simulink model "PID_controller_long"  (R2019a)
settings: Solver=VariableStepAuto  StartTime=0.0  StopTime=100  FixedStep=1e-3  RelTol=1e-5
values from neighbouring files (symbols this model uses):
  sys = ss(A,B,C,D,'StateName', {'u'; 'w'; 'q'; 'theta'; 'h'}, 'InputName', {'eta';'epsilon'})    [control_system_v01.m]    (also in control_system_v02.m = ss(A,B,C,D,'StateName', {'u'; 'w'; 'q'; 'theta'},          ')
undefined symbols (not defined in the file or in its folder): a, actuators, b, c, env, F, geometry, Light, MIL
libraries: simulink x2, hdlsllib x1, aerolibactuator x1, aerolibwind2 x1, dspmtrx3 x1
settings Model: Creator=tyson  LastModifiedBy=tyson
settings DebuggingCC: InheritedTsInSrcMsg=none

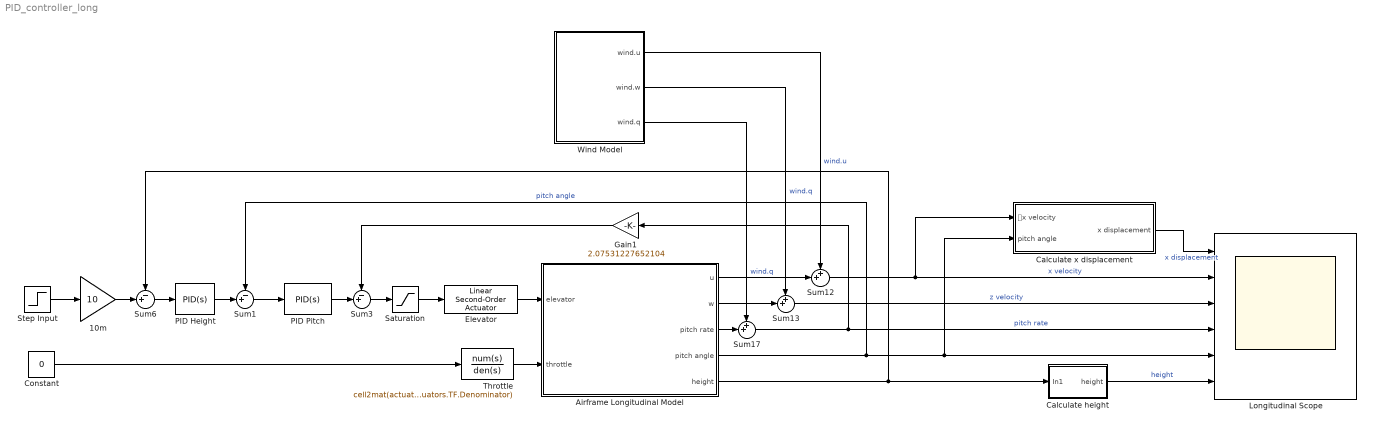
== system PID_controller_long ==
  10m : Gain  Gain=10
  Airframe Longitudinal Model : Subsystem
      mask Display: image('/home/tyson/Dropbox/Academic/4th Year/ELEN4011/matlab/icons/airframe_long.png');
  Calculate height : Subsystem
  Calculate x displacement : Subsystem
  Constant : Constant  Value=0
  Elevator : aerolibactuator/Linear Second-Order Actuator  wn_fin=actuators.naturalFreq  z_fin=actuators.dampingRatio  fin_act_0=0  fin_act_vel=0
      settings: SourceProductName=Aerospace Blockset  SourceProductBaseCode=AE
  Gain1 : Gain  Gain=2.07531227652104
  Longitudinal Scope : Scope  NumInputPorts=6
  PID Height : simulink/Continuous/PID Controller  Controller=PID  Form=Parallel  TimeDomain=Continuous-time  SampleTime=-1  IntegratorMethod=Forward Euler  FilterMethod=Forward Euler  ControllerParametersSource=internal  P=0.0203746551941326  I=3.98785899354423e-05  D=-0.014097541537027  UseFilter=on  N=1.21830283710381  TunerSelectOption=Transfer Function Based (PID Tuner App)  InitialConditionSource=internal  InitialConditionForIntegrator=0  InitialConditionForFilter=0  DifferentiatorICPrevScaledInput=0  ExternalReset=none  TrackingMode=off  Kt=1  LimitOutput=off  UpperSaturationLimit=deg2rad(12.5)  LowerSaturationLimit=-deg2rad(12.5)  LinearizeAsGain=on  AntiWindupMode=clamping  Kb=1  POutMin=[]  POutMax=[]  IOutMin=[]  IOutMax=[]  DOutMin=[]  DOutMax=[]  NOutMin=[]  NOutMax=[]  SumOutMin=[]  SumOutMax=[]  SaturationOutMin=[]  SaturationOutMax=[]  PParamMin=[]  PParamMax=[]  IParamMin=[]  IParamMax=[]  DParamMin=[]  DParamMax=[]  NParamMin=[]  NParamMax=[]  KbParamMin=[]  KbParamMax=[]  KtParamMin=[]  KtParamMax=[]  KbOutMin=[]  KbOutMax=[]  KtOutMin=[]  KtOutMax=[]  IntegratorOutMin=[]  IntegratorOutMax=[]  FilterOutMin=[]  FilterOutMax=[]  SumI1OutMin=[]  SumI1OutMax=[]  SumI2OutMin=[]  SumI2OutMax=[]  SumI3OutMin=[]  SumI3OutMax=[]  SumI4OutMin=[]  SumI4OutMax=[]  SumDOutMin=[]  SumDOutMax=[]  DifferentiatorOutMin=[]  DifferentiatorOutMax=[]  FilterDiffOutCoefMin=[]  FilterDiffOutCoefMax=[]  ReciprocalOutMin=[]  ReciprocalOutMax=[]  SumDenOutMin=[]  SumDenOutMax=[]  SumNumOutMin=[]  SumNumOutMax=[]  DivideOutMin=[]  DivideOutMax=[]  IntegratorContinuousStateAttributes=''  IntegratorStateMustResolveToSignalObject=off  IntegratorRTWStateStorageClass=Auto  FilterContinuousStateAttributes=''  FilterStateMustResolveToSignalObject=off  FilterRTWStateStorageClass=Auto  ParallelPVariant=InternalParameters  IdealPVariant=Disabled  IVariant=InternalParameters  DVariant=InternalParameters  IntegratorVariant=Continuous  SatVariant=Disabled  AWVariant=Passthrough  PCopyVariant=Disabled  TRVariant=Disabled  FdbkBlocksVariant=Forward  IdealPFdbkVariant=Disabled  SatFdbkVariant=Disabled  DerivativeFilterVariant=ContFilter  NVariant=InternalParameters  NCopyVariant=Disabled  FilterICVariant=InternalICsFilter  IntegratorICVariant=InternalICs  ExternalResetVariant=Disabled  TRSumVariant=Passthrough  SumFdbkVariant=Disabled  SumVariant=Sum_PID
  PID Pitch : simulink/Continuous/PID Controller  Controller=PID  Form=Parallel  TimeDomain=Continuous-time  SampleTime=-1  IntegratorMethod=Forward Euler  FilterMethod=Forward Euler  ControllerParametersSource=internal  P=11.4841294962751  I=3.73443810245113  D=6.13074519741651  UseFilter=on  N=502.258070962348  TunerSelectOption=Transfer Function Based (PID Tuner App)  InitialConditionSource=internal  InitialConditionForIntegrator=0  InitialConditionForFilter=0  DifferentiatorICPrevScaledInput=0  ExternalReset=none  TrackingMode=off  Kt=1  LimitOutput=on  UpperSaturationLimit=geometry.elevator.limits(1)  LowerSaturationLimit=geometry.elevator.limits(2)  LinearizeAsGain=on  AntiWindupMode=clamping  Kb=1  POutMin=[]  POutMax=[]  IOutMin=[]  IOutMax=[]  DOutMin=[]  DOutMax=[]  NOutMin=[]  NOutMax=[]  SumOutMin=[]  SumOutMax=[]  SaturationOutMin=[]  SaturationOutMax=[]  PParamMin=[]  PParamMax=[]  IParamMin=[]  IParamMax=[]  DParamMin=[]  DParamMax=[]  NParamMin=[]  NParamMax=[]  KbParamMin=[]  KbParamMax=[]  KtParamMin=[]  KtParamMax=[]  KbOutMin=[]  KbOutMax=[]  KtOutMin=[]  KtOutMax=[]  IntegratorOutMin=[]  IntegratorOutMax=[]  FilterOutMin=[]  FilterOutMax=[]  SumI1OutMin=[]  SumI1OutMax=[]  SumI2OutMin=[]  SumI2OutMax=[]  SumI3OutMin=[]  SumI3OutMax=[]  SumI4OutMin=[]  SumI4OutMax=[]  SumDOutMin=[]  SumDOutMax=[]  DifferentiatorOutMin=[]  DifferentiatorOutMax=[]  FilterDiffOutCoefMin=[]  FilterDiffOutCoefMax=[]  ReciprocalOutMin=[]  ReciprocalOutMax=[]  SumDenOutMin=[]  SumDenOutMax=[]  SumNumOutMin=[]  SumNumOutMax=[]  DivideOutMin=[]  DivideOutMax=[]  IntegratorContinuousStateAttributes=''  IntegratorStateMustResolveToSignalObject=off  IntegratorRTWStateStorageClass=Auto  FilterContinuousStateAttributes=''  FilterStateMustResolveToSignalObject=off  FilterRTWStateStorageClass=Auto  ParallelPVariant=InternalParameters  IdealPVariant=Disabled  IVariant=InternalParameters  DVariant=InternalParameters  IntegratorVariant=Continuous  SatVariant=Enabled  AWVariant=ContClampingParallel  PCopyVariant=Disabled  TRVariant=Disabled  FdbkBlocksVariant=Forward  IdealPFdbkVariant=Disabled  SatFdbkVariant=Disabled  DerivativeFilterVariant=ContFilter  NVariant=InternalParameters  NCopyVariant=Disabled  FilterICVariant=InternalICsFilter  IntegratorICVariant=InternalICs  ExternalResetVariant=Disabled  TRSumVariant=Passthrough  SumFdbkVariant=Disabled  SumVariant=Sum_PID
  Saturation : Saturate  UpperLimit=geometry.elevator.limits(1)  LowerLimit=geometry.elevator.limits(2)  LinearizeAsGain=off
  Step Input : Step  Time=0
  Sum1 : Sum  Inputs=-+|
  Sum12 : Sum  Inputs=++|
  Sum13 : Sum  Inputs=++|
  Sum17 : Sum  Inputs=++|
  Sum3 : Sum  Inputs=-+|
  Sum6 : Sum  Inputs=-+|
  Throttle : TransferFcn  Numerator=cell2mat(actuators.TF.Numerator)  Denominator=cell2mat(actuators.TF.Denominator)
  Wind Model : Subsystem
      mask Display: image('/home/tyson/Dropbox/Academic/4th Year/ELEN4011/matlab/icons/wind.png');
  wires:
  Airframe Longitudinal Model/4(pitch angle) -> Longitudinal Scope/5, Calculate x displacement/2(pitch angle), Sum1/1  "pitch angle"
  Sum13/1 -> Longitudinal Scope/3  "z velocity"
  Elevator/1 -> Airframe Longitudinal Model/1(elevator)
  Sum17/1 -> Longitudinal Scope/4, Gain1/1  "pitch rate"
  Sum1/1 -> PID Pitch/1
  PID Pitch/1 -> Sum3/2
  PID Height/1 -> Sum1/2
  Sum6/1 -> PID Height/1
  Sum3/1 -> Saturation/1
  Airframe Longitudinal Model/5(height) -> Calculate height/1(In1), Sum6/1
  Sum12/1 -> Calculate x displacement/1(𝚫x velocity), Longitudinal Scope/2  "x velocity"
  Calculate x displacement/1(x displacement) -> Longitudinal Scope/1  "x displacement"
  Airframe Longitudinal Model/1(u) -> Sum12/2
  Airframe Longitudinal Model/2(w) -> Sum13/2
  Airframe Longitudinal Model/3(pitch rate) -> Sum17/2
  Step Input/1 -> 10m/1
  10m/1 -> Sum6/2
  Wind Model/1(wind.u) -> Sum12/1  "wind.u"
  Wind Model/2(wind.w) -> Sum13/1  "wind.q"
  Wind Model/3(wind.q) -> Sum17/1  "wind.q"
  Throttle/1 -> Airframe Longitudinal Model/2(throttle)
  Gain1/1 -> Sum3/1
  Saturation/1 -> Elevator/1
  Constant/1 -> Throttle/1
  Calculate height/1(height) -> Longitudinal Scope/6  "height"

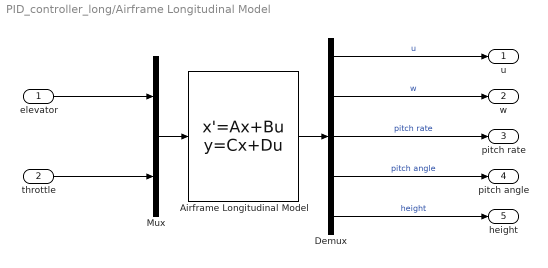
== system PID_controller_long/Airframe Longitudinal Model ==
  elevator : Inport
  throttle : Inport  Port=2
  Airframe Longitudinal Model : StateSpace  A=sys.long.A  B=sys.long.B  C=sys.long.C  D=sys.long.D  InitialCondition=0
  Demux : Demux  Outputs=5
  Mux : Mux  Inputs=2
  u : Outport
  w : Outport  Port=2
  pitch rate : Outport  Port=3
  pitch angle : Outport  Port=4
  height : Outport  Port=5
  wires:
  throttle/1 -> Mux/2
  Demux/4 -> pitch angle/1  "pitch angle"
  Demux/3 -> pitch rate/1  "pitch rate"
  Mux/1 -> Airframe Longitudinal Model/1
  Airframe Longitudinal Model/1 -> Demux/1
  Demux/1 -> u/1  "u"
  Demux/2 -> w/1  "w"
  Demux/5 -> height/1  "height"
  elevator/1 -> Mux/1

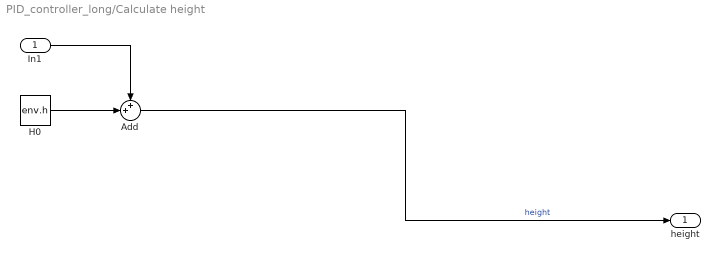
== system PID_controller_long/Calculate height ==
  In1 : Inport
  Add : Sum  Inputs=++|
  H0 : Constant  Value=env.h
  height : Outport
  wires:
  H0/1 -> Add/2
  In1/1 -> Add/1
  Add/1 -> height/1  "height"

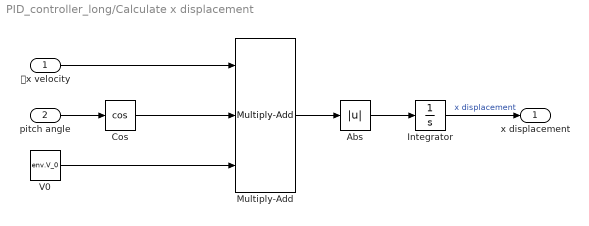
== system PID_controller_long/Calculate x displacement ==
  𝚫x velocity : Inport
  pitch angle : Inport  Port=2
  Abs : Abs
  Cos : Trigonometry  Operator=cos
  Integrator : Integrator
  Multiply-Add : hdlsllib/HDL Operations/Multiply-Add  Function=c+(a.*b)  datatype=Inherit: Inherit via internal rule  DoSatur=off  FMA=off
      settings: SourceProductName=Simulink  SourceProductBaseCode=SL
  V0 : Constant  Value=env.V_0
  x displacement : Outport
  wires:
  V0/1 -> Multiply-Add/3
  Abs/1 -> Integrator/1
  Cos/1 -> Multiply-Add/2
  pitch angle/1 -> Cos/1
  Integrator/1 -> x displacement/1  "x displacement"
  𝚫x velocity/1 -> Multiply-Add/1
  Multiply-Add/1 -> Abs/1

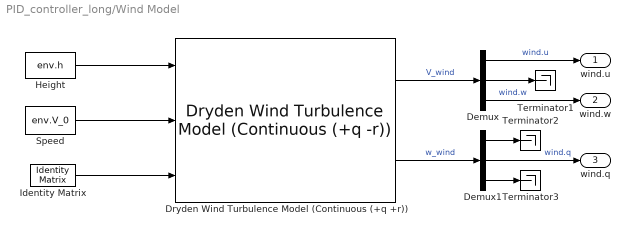
== system PID_controller_long/Wind Model ==
  Demux : Demux  Outputs=3
  Demux1 : Demux  Outputs=3
  Dryden Wind Turbulence Model (Continuous (+q +r)) : aerolibwind2/Dryden Wind Turbulence Model  (Continuous (+q -r))  units=Metric (MKS)  spec=MIL-F-8785C  model=Continuous Dryden (+q +r)  W20=10  Wdeg=0  TurbProb=10^-2 - Light  L_high=533.4  Wingspan=geometry.b  ts=0.1  Seed=[2341 2342 2343 2344]  T_on=on
      settings: SourceProductName=Aerospace Blockset
  Height : Constant  Value=env.h
  Identity Matrix : dspmtrx3/Identity Matrix  Inherit=off  N=3  Ts=1  dataType=double  isSigned=on  wordLen=16  udDataType=sfix(16)  fracBitsMode=Best precision  numFracBits=15  OutDataTypeStr=double  LastOutDataTypeStr=double
      settings: SourceProductName=DSP System Toolbox
  Speed : Constant  Value=env.V_0
  Terminator1 : Terminator
  Terminator2 : Terminator
  Terminator3 : Terminator
  wind.u : Outport
  wind.w : Outport  Port=2
  wind.q : Outport  Port=3
  wires:
  Demux/3 -> wind.w/1  "wind.w"
  Height/1 -> Dryden Wind Turbulence Model (Continuous (+q +r))/1
  Demux1/2 -> wind.q/1  "wind.q"
  Identity Matrix/1 -> Dryden Wind Turbulence Model (Continuous (+q +r))/3
  Dryden Wind Turbulence Model (Continuous (+q +r))/2 -> Demux1/1  "w_wind"
  Demux/2 -> Terminator1/1
  Demux/1 -> wind.u/1  "wind.u"
  Dryden Wind Turbulence Model (Continuous (+q +r))/1 -> Demux/1  "V_wind"
  Demux1/1 -> Terminator2/1
  Speed/1 -> Dryden Wind Turbulence Model (Continuous (+q +r))/2
  Demux1/3 -> Terminator3/1
